simulink model "non_linear"  (R2021a)
settings: Solver=VariableStepAuto  StartTime=0.0  StopTime=10.0  RelTol=1e-3
settings Model: Creator=vatsa  LastModifiedBy=vatsa

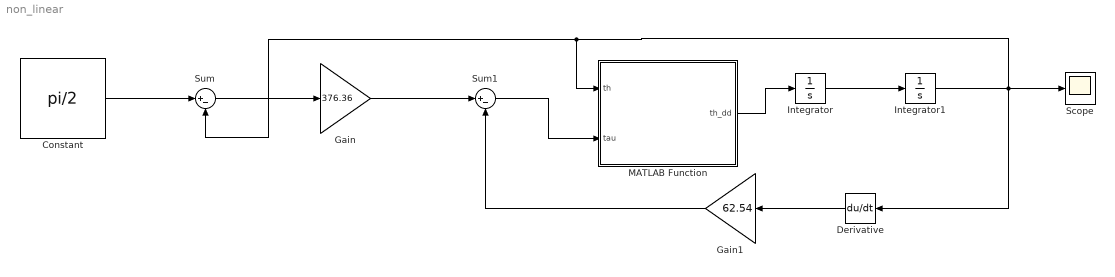
== system non_linear ==
  Constant : Constant  Value=pi/2
  Derivative : Derivative
  Gain : Gain  Gain=376.36
  Gain1 : Gain  Gain=62.54
  Integrator : Integrator
  Integrator1 : Integrator  InitialCondition=pi/4
  MATLAB Function : MATLAB Function  TreatAsAtomicUnit=on
  Scope : Scope
  Sum : Sum  Inputs=|+-
  Sum1 : Sum  Inputs=|+-
  wires:
  Constant/1 -> Sum/1
  Integrator/1 -> Integrator1/1
  MATLAB Function/1(th_dd) -> Integrator/1
  Sum/1 -> Gain/1
  Gain/1 -> Sum1/1
  Sum1/1 -> MATLAB Function/2(tau)
  Integrator1/1 -> Derivative/1, Scope/1, Sum/2, MATLAB Function/1(th)
  Gain1/1 -> Sum1/2
  Derivative/1 -> Gain1/1

== matlab function non_linear/MATLAB Function ==
  data: th input; th_dd output; tau input
function th_dd = fcn(th,tau)
g = 9.8;
l = 4;
m = 1;
th_dd = (sin(th)*(-g/l))+(tau/(m*l^2));
